simulink model "DCMotor_reduction"  (R2021a)
settings: Solver=VariableStepAuto  StartTime=0.0  StopTime=sim_time  MaxStep=step_size  RelTol=1e-3
values from neighbouring files (symbols this model uses):
  b = 3.5077E-6    (= 3.5077e-06)    [DCMotor_reduction_run.m]    (also in DCMotor_run.m; MassSpringDamper_run.m = 2; PID_ScriptOnly.m = 50; PID_SpringDamper_run.m = 10)
  J = 3.2284E-6    (= 3.2284e-06)    [DCMotor_reduction_run.m]    (also in DCMotor_run.m)
  Kb = 0.0274    [DCMotor_reduction_run.m]    (also in DCMotor_run.m)
  Kd = 0    [DCMotor_reduction_run.m]    (also in PID_SpringDamper_run.m = 50; PID_block_run.m; PID_vehicle_run.m)
  Ki = 1    [DCMotor_reduction_run.m]    (also in PID_ScriptOnly.m = 40; PID_SpringDamper_run.m = 300; PID_block_run.m = 0; PID_vehicle_run.m)
  Kp = 0.5    [DCMotor_reduction_run.m]    (also in PID_ScriptOnly.m = 800; PID_SpringDamper_run.m = 350; PID_block_run.m = 1000; PID_vehicle_run.m = 1)
  Kt = 0.0274    [DCMotor_reduction_run.m]    (also in DCMotor_run.m)
  L = 2.75E-6    (= 2.75e-06)    [DCMotor_reduction_run.m]    (also in DCMotor_run.m)
  R = 4    [DCMotor_reduction_run.m]    (also in DCMotor_run.m; OCV_PRC.m = 0.1)
  V = 1    [DCMotor_reduction_run.m]    (also in DCMotor_run.m; OCV_PRC.m = K0 - R * I(k) - K1/SOC - K2 * SOC + K3 * log(SOC) + K4 * log)
libraries: pid_lib x1
settings Model: Creator=shinyh  LastModifiedBy=shinyh

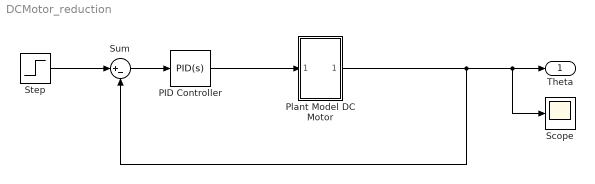
== system DCMotor_reduction ==
  PID Controller : pid_lib/PID Controller  Controller=PID  Form=Parallel  TimeDomain=Continuous-time  UseExternalTs=off  SampleTime=-1  IntegratorMethod=Forward Euler  FilterMethod=Forward Euler  ControllerParametersSource=internal  P=Kp  I=Ki  D=Kd  UseFilter=on  N=100  TunerSelectOption=Transfer Function Based (PID Tuner App)  InitialConditionSource=internal  InitialConditionForIntegrator=0  InitialConditionForFilter=0  DifferentiatorICPrevScaledInput=0  ExternalReset=none  TrackingMode=off  Kt=1  LimitOutput=off  SatLimitsSource=internal  UpperSaturationLimit=inf  LowerSaturationLimit=-inf  LinearizeAsGain=on  AntiWindupMode=none  Kb=1  POutMin=[]  POutMax=[]  IOutMin=[]  IOutMax=[]  DOutMin=[]  DOutMax=[]  NOutMin=[]  NOutMax=[]  SumOutMin=[]  SumOutMax=[]  SaturationOutMin=[]  SaturationOutMax=[]  PParamMin=[]  PParamMax=[]  IParamMin=[]  IParamMax=[]  DParamMin=[]  DParamMax=[]  NParamMin=[]  NParamMax=[]  KbParamMin=[]  KbParamMax=[]  KtParamMin=[]  KtParamMax=[]  KbOutMin=[]  KbOutMax=[]  KtOutMin=[]  KtOutMax=[]  IntegratorOutMin=[]  IntegratorOutMax=[]  FilterOutMin=[]  FilterOutMax=[]  SumI1OutMin=[]  SumI1OutMax=[]  SumI2OutMin=[]  SumI2OutMax=[]  SumI3OutMin=[]  SumI3OutMax=[]  SumI4OutMin=[]  SumI4OutMax=[]  SumDOutMin=[]  SumDOutMax=[]  DifferentiatorOutMin=[]  DifferentiatorOutMax=[]  FilterDiffOutCoefMin=[]  FilterDiffOutCoefMax=[]  ReciprocalOutMin=[]  ReciprocalOutMax=[]  SumDenOutMin=[]  SumDenOutMax=[]  SumNumOutMin=[]  SumNumOutMax=[]  DivideOutMin=[]  DivideOutMax=[]  UdiffTsProdOutMin=[]  UdiffTsProdOutMax=[]  NTsProdOutMin=[]  NTsProdOutMax=[]  UintegralTsProdOutMin=[]  UintegralTsProdOutMax=[]  UngainTsProdOutMin=[]  UngainTsProdOutMax=[]  IntegratorContinuousStateAttributes=''  IntegratorStateMustResolveToSignalObject=off  IntegratorRTWStateStorageClass=Auto  FilterContinuousStateAttributes=''  FilterStateMustResolveToSignalObject=off  FilterRTWStateStorageClass=Auto  ParallelPVariant=InternalParameters  IdealPVariant=Disabled  IVariant=InternalParameters  DVariant=InternalParameters  IntegratorVariant=Continuous  SatVariant=Disabled  AWVariant=Passthrough  PCopyVariant=Disabled  TRVariant=Disabled  FdbkBlocksVariant=Forward  IdealPFdbkVariant=Disabled  SatFdbkVariant=Disabled  DerivativeFilterVariant=ContFilter  NVariant=InternalParameters  NCopyVariant=Disabled  FilterICVariant=InternalICsFilter  IntegratorICVariant=InternalICs  ExternalResetVariant=Disabled  TRSumVariant=Passthrough  SumFdbkVariant=Disabled  SumVariant=Sum_PID  TsampFilterVariant=InternalTs  TsampNgainVariant=Passthrough  TsampIntegralVariant=Passthrough  ExternalSaturationOutDataTypeStr=Inherit: Same as second input
  Plant Model DC Motor : Subsystem
  Scope : Scope
  Step : Step  After=V  SampleTime=0
  Sum : Sum  Inputs=|+-
  Theta : Outport
  wires:
  Step/1 -> Sum/1
  Plant Model DC Motor/1(theta) -> Sum/2, Scope/1, Theta/1
  PID Controller/1 -> Plant Model DC Motor/1(In1)
  Sum/1 -> PID Controller/1

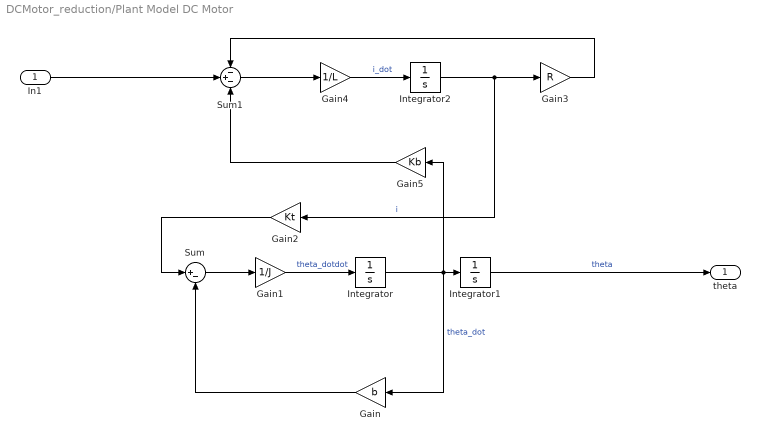
== system DCMotor_reduction/Plant Model DC Motor ==
  In1 : Inport
  Gain : Gain  Gain=b
  Gain1 : Gain  Gain=1/J
  Gain2 : Gain  Gain=Kt
  Gain3 : Gain  Gain=R
  Gain4 : Gain  Gain=1/L
  Gain5 : Gain  Gain=Kb
  Integrator : Integrator
  Integrator1 : Integrator
  Integrator2 : Integrator
  Sum : Sum  Inputs=|+-
  Sum1 : Sum  Inputs=-+-
  theta : Outport
  wires:
  Gain5/1 -> Sum1/3
  Integrator2/1 -> Gain3/1, Gain2/1  "i"
  Sum/1 -> Gain1/1
  Integrator/1 -> Gain5/1, Gain/1, Integrator1/1  "theta_dot"
  Gain/1 -> Sum/2
  Gain4/1 -> Integrator2/1  "i_dot"
  Integrator1/1 -> theta/1  "theta"
  Gain2/1 -> Sum/1
  Sum1/1 -> Gain4/1
  Gain1/1 -> Integrator/1  "theta_dotdot"
  Gain3/1 -> Sum1/1
  In1/1 -> Sum1/2
